simulink model "openLoopTestBed"  (Simulink 8.6)
settings: Solver=VariableStepAuto  SolverMode=SingleTasking  StartTime=0.0  StopTime=10.0  FixedStep=Ts  MaxStep=0.1  RelTol=1e-3
values from neighbouring files (symbols this model uses):
  Ts = 0.01    [conductOpenLoopTestonVirtualPlant.m]    (also in sineSweepOnVirtualPlant.m = 1/Fs)
settings Model: Creator=pbarooah  LastModifiedBy=pbarooah
settings DataIOCC: ExternalInput=u  LimitDataPoints=off  SaveFormat=Dataset  SignalLoggingSaveFormat=Dataset
settings OptimizationCC: ExpressionDepthLimit=128
settings DebuggingCC: UnderspecifiedInitializationDetection=Simplified  MergeDetectMultiDrivingBlocksExec=error  SolverPrmCheckMsg=none  FcnCallInpInsideContextMsg=EnableAllAsError  AllowSymbolicDim=on  StateNameClashWarn=none  SFUnexpectedBacktrackingDiag=error  SFNoUnconditionalDefaultTransitionDiag=error
settings HardwareCC: ProdBitPerPointer=64  ProdLargestAtomicFloat=Float  ProdIntDivRoundTo=Zero  ProdEndianess=LittleEndian  ProdWordSize=64  ProdHWDeviceType=Intel->x86-64 (Windows64)
settings ModelReferenceCC: PropagateSignalLabelsOutOfModel=on
settings GRTTargetCC: TargetLangStandard=C99 (ISO)  GeneratePreprocessorConditionals=Use local settings  CombineOutputUpdateFcns=on  GRTInterface=off
settings ConfigComp: CovMetricSettings=dwe  CovHtmlReporting=off  CovSaveCumulativeToWorkspaceVar=off  CovSaveSingleToWorkspaceVar=off  CovExternalEMLEnable=on

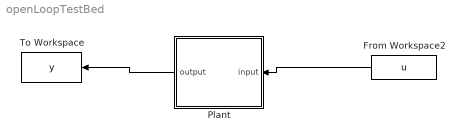
== system openLoopTestBed ==
  From Workspace2 : FromWorkspace  VariableName=u  SampleTime=Ts
  "Plant " : Subsystem
  To Workspace : ToWorkspace  VariableName=y  SaveFormat=Structure With Time  SampleTime=Ts
  wires:
  "Plant "/1(output) -> To Workspace/1
  From Workspace2/1 -> "Plant "/1(input)

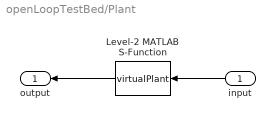
== system openLoopTestBed/Plant  ==
  input : Inport
  Level-2 MATLAB S-Function : M-S-Function  FunctionName=virtualPlant
  output : Outport
  wires:
  input/1 -> Level-2 MATLAB S-Function/1
  Level-2 MATLAB S-Function/1 -> output/1
